simulink model "task2"  (Simulink 7.5)
settings: Solver=ode45  StartTime=0.0  StopTime=0.4  RelTol=1e-3
settings Model: Creator=Dranik_win  LastModifiedBy=Dranik_win

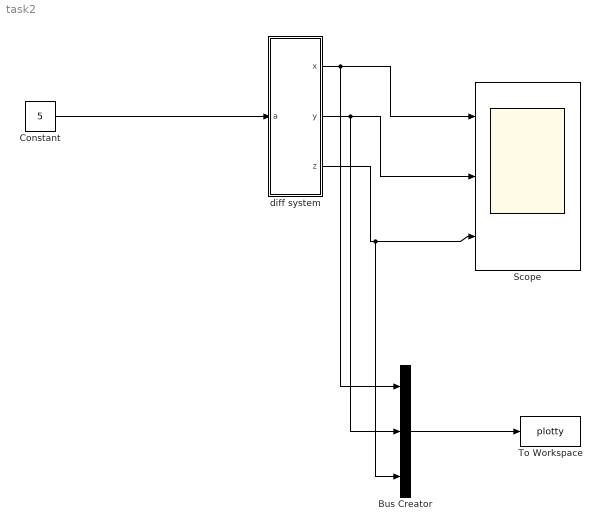
== system task2 ==
  Bus Creator : BusCreator  Inputs=3
  Constant : Constant  Value=5  OutDataType=fixdt(1, 16)  OutScaling=2^0
  Scope : Scope  NumInputPorts=3
      settings: YMin=-5~-5~-5  YMax=5~5~5
  To Workspace : ToWorkspace  VariableName=plotty  SampleTime=-1  SaveFormat=Array
  diff system : Subsystem
  wires:
  Constant/1 -> diff system/1(a)
  diff system/1(x) -> Scope/1, Bus Creator/1
  diff system/2(y) -> Scope/2, Bus Creator/2
  diff system/3(z) -> Scope/3, Bus Creator/3
  Bus Creator/1 -> To Workspace/1

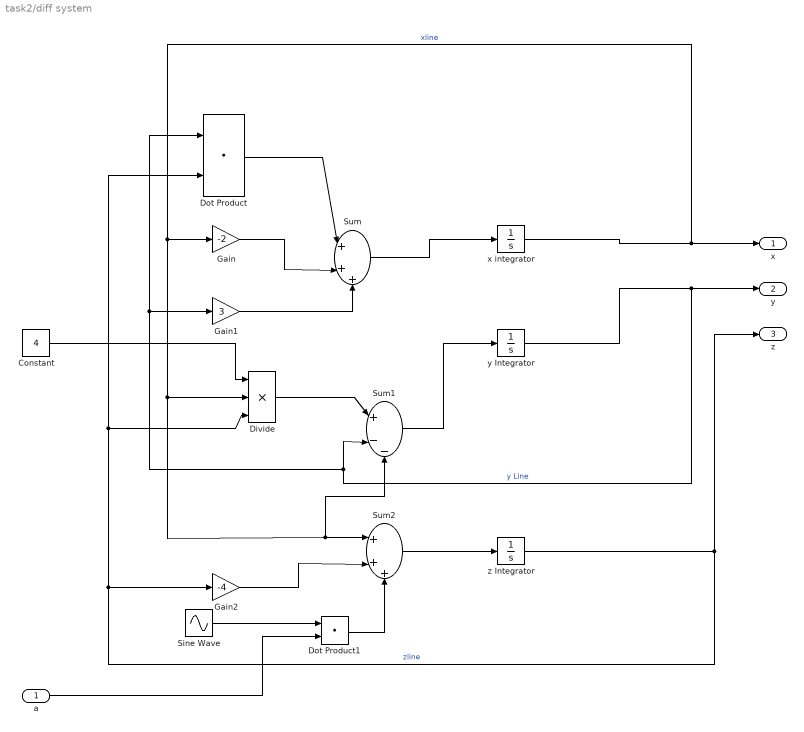
== system task2/diff system ==
  a : Inport  OutDataType=fixdt(1, 16)  OutScaling=2^0
  Constant : Constant  Value=4  OutDataType=fixdt(1, 16)  OutScaling=2^0
  Divide : Product  Inputs=***  OutDataType=fixdt(1, 16)  OutScaling=2^-10
  Dot Product : DotProduct  OutDataType=fixdt(1, 16)  OutScaling=2^-10  InputSameDT=on  OutDataTypeStr=Inherit: Inherit via internal rule
  Dot Product1 : DotProduct  OutDataType=fixdt(1, 16)  OutScaling=2^-10  InputSameDT=on  OutDataTypeStr=Inherit: Inherit via internal rule
  Gain : Gain  Gain=-2  ParameterDataType=fixdt(1, 16)  ParameterScaling=2^0  OutDataType=fixdt(1, 16)  OutScaling=2^0
  Gain1 : Gain  Gain=3  ParameterDataType=fixdt(1, 16)  ParameterScaling=2^0  OutDataType=fixdt(1, 16)  OutScaling=2^0
  Gain2 : Gain  Gain=-4  ParameterDataType=fixdt(1, 16)  ParameterScaling=2^0  OutDataType=fixdt(1, 16)  OutScaling=2^0
  Sine Wave : Sin  Amplitude=1  Bias=0  Frequency=4  Phase=pi/2  Samples=10  SampleTime=0  Offset=0
  Sum : Sum  Inputs=|+++  OutDataType=fixdt(1, 16)  OutScaling=2^0
  Sum1 : Sum  Inputs=|+--  OutDataType=fixdt(1, 16)  OutScaling=2^0
  Sum2 : Sum  Inputs=|+++  OutDataType=fixdt(1, 16)  OutScaling=2^0
  x integrator : Integrator  InitialCondition=3
  y Integrator : Integrator  InitialCondition=4
  z Integrator : Integrator  InitialCondition=4
  x : Outport  OutDataType=fixdt(1, 16)  OutScaling=2^0
  y : Outport  Port=2  OutDataType=fixdt(1, 16)  OutScaling=2^0
  z : Outport  Port=3  OutDataType=fixdt(1, 16)  OutScaling=2^0
  wires:
  Dot Product1/1 -> Sum2/3
  Sine Wave/1 -> Dot Product1/1
  a/1 -> Dot Product1/2
  Gain2/1 -> Sum2/2
  z Integrator/1 -> Dot Product/2, Divide/3, Gain2/1, z/1  "zline"
  Sum2/1 -> z Integrator/1
  y Integrator/1 -> y/1, Sum1/2, Gain1/1, Dot Product/1  "y Line"
  Sum1/1 -> y Integrator/1
  Divide/1 -> Sum1/1
  Constant/1 -> Divide/1
  x integrator/1 -> Gain/1, Divide/2, Sum2/1, Sum1/3, x/1  "xline"
  Sum/1 -> x integrator/1
  Gain1/1 -> Sum/3
  Dot Product/1 -> Sum/1
  Gain/1 -> Sum/2
